simulink model "Lab1_7B"  (R2018a)
settings: Solver=VariableStepAuto  StartTime=0.0  StopTime=30  RelTol=1e-3
settings Model: Creator=melab2  LastModifiedBy=rahul

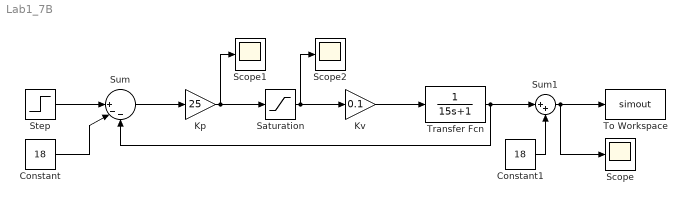
== system Lab1_7B ==
  Constant : Constant  Value=18
  Constant1 : Constant  Value=18
  Kp : Gain  Gain=25
  Kv : Gain  Gain=0.1
  Saturation : Saturate  UpperLimit=25  LowerLimit=-75
  Scope : Scope
  Scope1 : Scope
  Scope2 : Scope
  Step : Step  Before=18  After=17  SampleTime=0
  Sum : Sum  Inputs=||+--
  Sum1 : Sum  Inputs=|++
  To Workspace : ToWorkspace  VariableName=simout  SampleTime=-1
  Transfer Fcn : TransferFcn  Denominator=[15 1]
  wires:
  Sum/1 -> Kp/1
  Kv/1 -> Transfer Fcn/1
  Step/1 -> Sum/1
  Kp/1 -> Scope1/1, Saturation/1
  Saturation/1 -> Scope2/1, Kv/1
  Constant/1 -> Sum/2
  Transfer Fcn/1 -> Sum/3, Sum1/1
  Sum1/1 -> Scope/1, To Workspace/1
  Constant1/1 -> Sum1/2
